simulink model "Target_Control_System"  (R2021b)
settings: Solver=FixedStepDiscrete  StartTime=0.0  StopTime=5  RelTol=1e-3
PreLoadFcn:
  | RTWConfigurationCB('preloadfcn', bdroot);
PostLoadFcn:
  | load('configuration/data_struct.mat');
  | load('configuration/fluxMaps_propMotor.mat');
  | load('configuration/parameterInit_PROP.mat');
  | load('configuration/parameterInit_PUMP.mat');
  | load('configuration/parameterInit_PITCH.mat');
  | load('configuration/parameterInit_TILT.mat');
  | %load('configuration/base_workspace_signal_definition.mat');
  | %load('resolvedatastores_to_baseworkspace_for_faster_simulation.mat');
model workspace (MAT data in the model file):
  SIMULATION_OPTIONS : Simulink.Parameter (value not decoded)
  TARGET_CODE_GEN : Simulink.Parameter (value not decoded)
  TCS_SAMPLE_FREQ_HZ : Simulink.Parameter (value not decoded)
symbols that are objects in the model workspace (value not decoded): TARGET_CODE_GEN, TCS_SAMPLE_FREQ_HZ
undefined symbols (not defined in the file): A_DQ_REF_LPF_INIT__PITCH, A_DQ_REF_LPF_INIT__PROP, A_DQ_REF_LPF_INIT__PUMP, A_DQ_REF_LPF_INIT__TILT, A_OBSERVER_CONFIDENCE_INIT__PITCH, A_OBSERVER_CONFIDENCE_INIT__PROP, A_OBSERVER_CONFIDENCE_INIT__PUMP, A_OBSERVER_CONFIDENCE_INIT__TILT, ACTUATOR_MAX_ANGLE_TRIP__PITCH, ACTUATOR_MIN_ANGLE_TRIP__PITCH, ACTUATOR_POS_SENSOR_INV_DIRECTION__PITCH, ACTUATOR_POS_SENSOR_INV_DIRECTION__TILT, ACTUATOR_POS_SENSOR_OFFSET__PITCH, ACTUATOR_POS_SENSOR_OFFSET__TILT, ADC_scaler1_baseaddr_TILT, ADC_SCALER_FLOAT_TO_FIXPOINT_EXPANSION, ANGLE_ELEC_FROM_SENSOR_OFFSET_INIT__PITCH, ANGLE_ELEC_FROM_SENSOR_OFFSET_INIT__PROP, ANGLE_ELEC_FROM_SENSOR_OFFSET_INIT__PUMP, ANGLE_ELEC_FROM_SENSOR_OFFSET_INIT__TILT, AUTO_CLEAR_FAULTS_ENABLED__PITCH, AUTO_CLEAR_FAULTS_ENABLED__PROP, AUTO_CLEAR_FAULTS_ENABLED__PUMP, AUTO_CLEAR_FAULTS_ENABLED__TILT, AUTO_CLEAR_FAULTS_WAIT_TICKS__PITCH, AUTO_CLEAR_FAULTS_WAIT_TICKS__PROP, AUTO_CLEAR_FAULTS_WAIT_TICKS__PUMP, AUTO_CLEAR_FAULTS_WAIT_TICKS__TILT, AUTO_I_ZERO_IDLE_TICKS__PITCH, AUTO_I_ZERO_IDLE_TICKS__PROP, AUTO_I_ZERO_IDLE_TICKS__PUMP, AUTO_I_ZERO_IDLE_TICKS__TILT, AUTO_I_ZERO_OFFSET_IDC_THRESHOLD__PITCH, AUTO_I_ZERO_OFFSET_IDC_THRESHOLD__PROP, AUTO_I_ZERO_OFFSET_IDC_THRESHOLD__PUMP, AUTO_I_ZERO_OFFSET_IDC_THRESHOLD__TILT, AUTO_I_ZERO_OFFSET_IPH_THRESHOLD__PITCH, AUTO_I_ZERO_OFFSET_IPH_THRESHOLD__PROP, AUTO_I_ZERO_OFFSET_IPH_THRESHOLD__PUMP, AUTO_I_ZERO_OFFSET_IPH_THRESHOLD__TILT, AUTO_SENSORLESS_SWITCHOVER_DISABLE_OMEGA, AUTO_SENSORLESS_SWITCHOVER_ENABLE_OMEGA, AUTO_SENSORLESS_SWITCHOVER_MIN_CONFIDENCE, AUXILIARY_PROTECTION_UNIT_BASEADDR__TILT, blanking_max_error_omega_INIT_PITCH, blanking_max_error_omega_INIT_TILT, blanking_max_error_position_INIT_PITCH, blanking_max_error_position_INIT_TILT, BRUTE_START_I_Q_REF_RAMP_SPEED__PITCH, BRUTE_START_I_Q_REF_RAMP_SPEED__PROP, BRUTE_START_I_Q_REF_RAMP_SPEED__PUMP, BRUTE_START_I_Q_REF_RAMP_SPEED__TILT, CONTROL_LOOP_DT_INIT__PITCH, CONTROL_LOOP_DT_INIT__PROP, CONTROL_LOOP_DT_INIT__PUMP, CONTROL_LOOP_DT_INIT__TILT, CORRECTION_FILTER_SCALE__PITCH, CORRECTION_FILTER_SCALE__PROP, CORRECTION_FILTER_SCALE__PUMP, CORRECTION_FILTER_SCALE__TILT ... (+458)
libraries: simulink x178, Reusables_Lib x24
(part 15 of 47)

== system Target_Control_System/Target_Control_System/MainLoop/pumpMotor_mainLoop/motorTaskMainFastStep(&oPump)/Lowpass Filtered Quantities for External World - Pump ==
  note: Low-pass filtered quantities for external world
  lpfQuantities : TriggerPort  TriggerType=function-call  VariantControl=Variant
  Constant1 : Constant  Value=0.00008  OutDataTypeStr=single  SampleTime=-1
  Data Store Read101 : DataStoreRead  DataStoreName=oPump  DataStoreElements=oPump.oMot_.oOut_.fIdLpf_  IndexOptions=Index vector (dialog)  Indices=1  OutputSizes=1
  Data Store Read102 : DataStoreRead  DataStoreName=oPump  DataStoreElements=oPump.oMot_.oOut_.fIqLpf_  IndexOptions=Index vector (dialog)  Indices=1  OutputSizes=1
  Data Store Read103 : DataStoreRead  DataStoreName=oPump  DataStoreElements=oPump.oMot_.oIn_.oAdcData_.fUdc_  IndexOptions=Index vector (dialog)  Indices=1  OutputSizes=1
  Data Store Read107 : DataStoreRead  DataStoreName=oPump  DataStoreElements=oPump.oMot_.oOut_.fUdcLpf_  IndexOptions=Index vector (dialog)  Indices=1  OutputSizes=1
  Data Store Read108 : DataStoreRead  DataStoreName=oPump  DataStoreElements=oPump.oMot_.oIn_.oAdcData_.fIdc_  IndexOptions=Index vector (dialog)  Indices=1  OutputSizes=1
  Data Store Read109 : DataStoreRead  DataStoreName=oPump  DataStoreElements=oPump.oMot_.oOut_.fIdcLpf_  IndexOptions=Index vector (dialog)  Indices=1  OutputSizes=1
  Data Store Read110 : DataStoreRead  DataStoreName=oPump  DataStoreElements=oPump.oMot_.oIn_.fPowerDc_  IndexOptions=Index vector (dialog)  Indices=1  OutputSizes=1
  Data Store Read111 : DataStoreRead  DataStoreName=oPump  DataStoreElements=oPump.oMot_.oOut_.fPowerDcLpf_  IndexOptions=Index vector (dialog)  Indices=1  OutputSizes=1
  Data Store Read112 : DataStoreRead  DataStoreName=oPump  DataStoreElements=oPump.oMot_.oOut_.fTEstimateLpf_  IndexOptions=Index vector (dialog)  Indices=1  OutputSizes=1
  Data Store Read113 : DataStoreRead  DataStoreName=oPump  DataStoreElements=oPump.oMot_.oState_.oRampDataIqRef_.fRampOut_  IndexOptions=Index vector (dialog)  Indices=1  OutputSizes=1
  Data Store Read114 : DataStoreRead  DataStoreName=oPump  DataStoreElements=oPump.oMot_.oOut_.fIqRefRampOutLpf_  IndexOptions=Index vector (dialog)  Indices=1  OutputSizes=1
  Data Store Read115 : DataStoreRead  DataStoreName=oPump  DataStoreElements=oPump.oMot_.oParam_.fADqRefLpf_  IndexOptions=Index vector (dialog)  Indices=1  OutputSizes=1
  Data Store Read116 : DataStoreRead  DataStoreName=oPump  DataStoreElements=oPump.oMot_.oIn_.fIdRefTotal_  IndexOptions=Index vector (dialog)  Indices=1  OutputSizes=1
  Data Store Read117 : DataStoreRead  DataStoreName=oPump  DataStoreElements=oPump.oMot_.oOut_.fIdRefLpf_  IndexOptions=Index vector (dialog)  Indices=1  OutputSizes=1
  Data Store Read118 : DataStoreRead  DataStoreName=oPump  DataStoreElements=oPump.oMot_.oIn_.fUqRef_  IndexOptions=Index vector (dialog)  Indices=1  OutputSizes=1
  Data Store Read119 : DataStoreRead  DataStoreName=oPump  DataStoreElements=oPump.oMot_.oOut_.fUqRefLpf_  IndexOptions=Index vector (dialog)  Indices=1  OutputSizes=1
  Data Store Read120 : DataStoreRead  DataStoreName=oPump  DataStoreElements=oPump.oMot_.oIn_.fUdRef_  IndexOptions=Index vector (dialog)  Indices=1  OutputSizes=1
  Data Store Read121 : DataStoreRead  DataStoreName=oPump  DataStoreElements=oPump.oMot_.oOut_.fUdRefLpf_  IndexOptions=Index vector (dialog)  Indices=1  OutputSizes=1
  Data Store Read17 : DataStoreRead  DataStoreName=oPump  DataStoreElements=oPump.oMot_.oIn_.fId_  IndexOptions=Index vector (dialog)  Indices=1  OutputSizes=1
  Data Store Read24 : DataStoreRead  DataStoreName=oPump  DataStoreElements=oPump.oMot_.oIn_.fIq_  IndexOptions=Index vector (dialog)  Indices=1  OutputSizes=1
  Data Store Read53 : DataStoreRead  DataStoreName=oPump  DataStoreElements=oPump.oMot_.oIn_.fTEstimate_  IndexOptions=Index vector (dialog)  Indices=1  OutputSizes=1
  Data Store Read88 : DataStoreRead  DataStoreName=oPump  DataStoreElements=oPump.oMot_.oOut_.fPowerDcLpf_  IndexOptions=Index vector (dialog)  Indices=1  OutputSizes=1
  Data Store Read89 : DataStoreRead  DataStoreName=oPump  DataStoreElements=oPump.oMot_.oOut_.fPowerDcXlpf_  IndexOptions=Index vector (dialog)  Indices=1  OutputSizes=1
  Data Store Read90 : DataStoreRead  DataStoreName=oPump  DataStoreElements=oPump.oMot_.oIn_.fOmegaEObserverLpf2_  IndexOptions=Index vector (dialog)  Indices=1  OutputSizes=1
  Data Store Read91 : DataStoreRead  DataStoreName=oPump  DataStoreElements=oPump.oMot_.oOut_.fOmegaEObserverXlpf2_  IndexOptions=Index vector (dialog)  Indices=1  OutputSizes=1
  Data Store Read96 : DataStoreRead  DataStoreName=oPump  DataStoreElements=oPump.oMot_.oParam_.fAOmegaXfilter2_  IndexOptions=Index vector (dialog)  Indices=1  OutputSizes=1
  Data Store Read97 : DataStoreRead  DataStoreName=oPump  DataStoreElements=oPump.oMot_.oParam_.fSlowPassFactor_  IndexOptions=Index vector (dialog)  Indices=1  OutputSizes=1
  Data Store Read98 : DataStoreRead  DataStoreName=oPump  DataStoreElements=oPump.oMot_.oIn_.fIPhaseMagnitude_  IndexOptions=Index vector (dialog)  Indices=1  OutputSizes=1
  Data Store Read99 : DataStoreRead  DataStoreName=oPump  DataStoreElements=oPump.oMot_.oState_.fIPhaseMagnitudeLpf_  IndexOptions=Index vector (dialog)  Indices=1  OutputSizes=1
  Data Store Write2 : DataStoreWrite  DataStoreName=oPump  DataStoreElements=oPump.oMot_.oOut_.fPowerDcXlpf_  IndexOptions=Index vector (dialog)  Indices=1  OutputSizes=1
  Data Store Write29 : DataStoreWrite  DataStoreName=oPump  DataStoreElements=oPump.oMot_.oOut_.fIdLpf_  IndexOptions=Index vector (dialog)  Indices=1  OutputSizes=1
  Data Store Write3 : DataStoreWrite  DataStoreName=oPump  DataStoreElements=oPump.oMot_.oState_.fIPhaseMagnitudeLpf_  IndexOptions=Index vector (dialog)  Indices=1  OutputSizes=1
  Data Store Write34 : DataStoreWrite  DataStoreName=oPump  DataStoreElements=oPump.oMot_.oOut_.fIqLpf_  IndexOptions=Index vector (dialog)  Indices=1  OutputSizes=1
  Data Store Write37 : DataStoreWrite  DataStoreName=oPump  DataStoreElements=oPump.oMot_.oOut_.fUdcLpf_  IndexOptions=Index vector (dialog)  Indices=1  OutputSizes=1
  Data Store Write38 : DataStoreWrite  DataStoreName=oPump  DataStoreElements=oPump.oMot_.oOut_.fIdcLpf_  IndexOptions=Index vector (dialog)  Indices=1  OutputSizes=1
  Data Store Write39 : DataStoreWrite  DataStoreName=oPump  DataStoreElements=oPump.oMot_.oOut_.fPowerDcLpf_  IndexOptions=Index vector (dialog)  Indices=1  OutputSizes=1
  Data Store Write40 : DataStoreWrite  DataStoreName=oPump  DataStoreElements=oPump.oMot_.oOut_.fTEstimateLpf_  IndexOptions=Index vector (dialog)  Indices=1  OutputSizes=1
  Data Store Write41 : DataStoreWrite  DataStoreName=oPump  DataStoreElements=oPump.oMot_.oOut_.fOmegaEObserverXlpf2_  IndexOptions=Index vector (dialog)  Indices=1  OutputSizes=1
  Data Store Write42 : DataStoreWrite  DataStoreName=oPump  DataStoreElements=oPump.oMot_.oOut_.fIqRefRampOutLpf_  IndexOptions=Index vector (dialog)  Indices=1  OutputSizes=1
  Data Store Write45 : DataStoreWrite  DataStoreName=oPump  DataStoreElements=oPump.oMot_.oOut_.fIdRefLpf_  IndexOptions=Index vector (dialog)  Indices=1  OutputSizes=1
  Data Store Write46 : DataStoreWrite  DataStoreName=oPump  DataStoreElements=oPump.oMot_.oOut_.fUqRefLpf_  IndexOptions=Index vector (dialog)  Indices=1  OutputSizes=1
  Data Store Write47 : DataStoreWrite  DataStoreName=oPump  DataStoreElements=oPump.oMot_.oOut_.fUdRefLpf_  IndexOptions=Index vector (dialog)  Indices=1  OutputSizes=1
  Divide{8..20} (13 alike) : Product  Inputs=**
  Sum{4..5,7,10..11,13,15,18,20..22,25,29} (13 alike) : Sum  Inputs=|+-
  Sum{3,6,8..9,12,14,16..17,19,24,26,30..31} (13 alike) : Sum  Inputs=|++
  wires:
  Data Store Read89/1 -> Sum24/2, Sum21/2
  Data Store Read117/1 -> Sum20/2, Sum19/2
  Sum10/1 -> Divide13/2
  Data Store Read98/1 -> Sum7/1
  Divide19/1 -> Sum31/1
  Data Store Read119/1 -> Sum29/2, Sum30/2
  Sum15/1 -> Divide14/2
  Sum30/1 -> Data Store Write46/1
  Data Store Read88/1 -> Sum21/1
  Data Store Read121/1 -> Sum25/2, Sum31/2
  Data Store Read116/1 -> Sum20/1
  Divide8/1 -> Sum3/1
  Sum7/1 -> Divide8/2
  Sum20/1 -> Divide16/2
  Data Store Read110/1 -> Sum11/1
  Divide9/1 -> Sum6/1
  Data Store Read111/1 -> Sum14/2, Sum11/2
  Sum21/1 -> Divide20/2
  Sum25/1 -> Divide19/2
  Sum29/1 -> Divide17/2
  Sum5/1 -> Divide10/2
  Data Store Read115/1 -> Divide15/1, Divide16/1, Divide19/1, Divide17/1
  Sum11/1 -> Divide11/2
  Data Store Read109/1 -> Sum12/2, Sum10/2
  Sum31/1 -> Data Store Write47/1
  Divide15/1 -> Sum17/1
  Data Store Read108/1 -> Sum10/1
  Divide18/1 -> Sum26/1
  Data Store Read99/1 -> Sum7/2, Sum3/2
  Sum8/1 -> Data Store Write34/1
  Sum13/1 -> Divide12/2
  Data Store Read97/1 -> Divide8/1, Divide9/1, Divide10/1, Divide12/1, Divide13/1, Divide14/1, Divide11/1
  Sum3/1 -> Data Store Write3/1
  Sum26/1 -> Data Store Write41/1
  Sum6/1 -> Data Store Write29/1
  Data Store Read112/1 -> Sum16/2, Sum15/2
  Divide17/1 -> Sum30/1
  Data Store Read90/1 -> Sum22/1
  Sum14/1 -> Data Store Write39/1
  Data Store Read102/1 -> Sum5/2, Sum8/2
  Data Store Read118/1 -> Sum29/1
  Sum9/1 -> Data Store Write37/1
  Sum18/1 -> Divide15/2
  Divide14/1 -> Sum16/1
  Sum22/1 -> Divide18/2
  Sum19/1 -> Data Store Write45/1
  Sum4/1 -> Divide9/2
  Sum12/1 -> Data Store Write38/1
  Data Store Read120/1 -> Sum25/1
  Sum17/1 -> Data Store Write42/1
  Divide12/1 -> Sum9/1
  Data Store Read91/1 -> Sum26/2, Sum22/2
  Divide10/1 -> Sum8/1
  Constant1/1 -> Divide20/1
  Data Store Read17/1 -> Sum4/1
  Data Store Read107/1 -> Sum9/2, Sum13/2
  Divide13/1 -> Sum12/1
  Data Store Read113/1 -> Sum18/1
  Data Store Read53/1 -> Sum15/1
  Data Store Read24/1 -> Sum5/1
  Divide20/1 -> Sum24/1
  Data Store Read103/1 -> Sum13/1
  Data Store Read101/1 -> Sum4/2, Sum6/2
  Data Store Read96/1 -> Divide18/1
  Divide16/1 -> Sum19/1
  Data Store Read114/1 -> Sum18/2, Sum17/2
  Sum24/1 -> Data Store Write2/1
  Sum16/1 -> Data Store Write40/1
  Divide11/1 -> Sum14/1

== system Target_Control_System/Target_Control_System/MainLoop/pumpMotor_mainLoop/motorTaskMainFastStep(&oPump)/Observer Confidence - Pump ==
  note: Observer confidence
      | // Two contributions, each adding 1/3 to give a value in range 0.0-1.0:
      | 	//  1. Magnitude of estimated flux relative to nominal flux (perhaps not for induction motors)
      | 	//  2. The relative noise on the estimated speed
  observerConfidence : TriggerPort  TriggerType=function-call  VariantControl=Variant
  Abs2 : Abs  OutDataTypeStr=single
  Abs3 : Abs  OutDataTypeStr=single
  Abs5 : Abs  OutDataTypeStr=single
  Add10 : Sum  Inputs=|-+
  Add11 : Sum
  Add2 : Sum  Inputs=+-
  Add7 : Sum  Inputs=|+-
  Add8 : Sum  Inputs=|-+
  Add9 : Sum  Inputs=|-+
  Constant14 : Constant  OutDataTypeStr=single  SampleTime=-1
  Data Store Read1 : DataStoreRead  DataStoreName=oPump  DataStoreElements=oPump.oMot_.oParam_.fAObserverConfidence_  IndexOptions=Index vector (dialog)  Indices=1  OutputSizes=1
  Data Store Read37 : DataStoreRead  DataStoreName=oPump  DataStoreElements=oPump.oMot_.oIn_.fOmegaEObserverLpf2_  IndexOptions=Index vector (dialog)  Indices=1  OutputSizes=1
  Data Store Read4 : DataStoreRead  DataStoreName=oPump  DataStoreElements=oPump.oMot_.oIn_.fFluxMainMagnitudeLpf_  IndexOptions=Index vector (dialog)  Indices=1  OutputSizes=1
  Data Store Read61 : DataStoreRead  DataStoreName=oPump  DataStoreElements=oPump.oMot_.oIn_.fOmegaEObserverRaw2_  IndexOptions=Index vector (dialog)  Indices=1  OutputSizes=1
  Data Store Read83 : DataStoreRead  DataStoreName=oPump  DataStoreElements=oPump.oMot_.oParam_.fMainFluxNominal_  IndexOptions=Index vector (dialog)  Indices=1  OutputSizes=1
  Data Store Write33 : DataStoreWrite  DataStoreName=oPump  DataStoreElements=oPump.oMot_.oState_.fObserverConfidence_  IndexOptions=Index vector (dialog)  Indices=1  OutputSizes=1
  Divide1 : Product  Inputs=*/
  Divide2 : Product  Inputs=*/
  Gain11 : Gain  Gain=0.83
  Gain5 : Gain  Gain=0.4
  Half : Constant  Value=0.5  OutDataTypeStr=single  SampleTime=-1
  Half1 : Constant  Value=0.5  OutDataTypeStr=single  SampleTime=-1
  IIR : Subsystem
  Saturation2 : Saturate  UpperLimit=1.25  LowerLimit=-inf
  Saturation3 : Saturate  UpperLimit=0.6  LowerLimit=-inf
  Switch3 : Switch  Criteria=u2 > Threshold  Threshold=0.5
  Zero0 : Constant  Value=0  OutDataTypeStr=single  SampleTime=-1
  isNaN : RelationalOperator  Operator=isNaN  OutDataTypeStr=boolean  RndMeth=Simplest
  wires:
  Saturation2/1 -> Gain5/1
  Switch3/1 -> IIR/1(In)
  Data Store Read4/1 -> Add7/1
  Half1/1 -> Add10/2
  Saturation3/1 -> Gain11/1
  Constant14/1 -> Add2/1
  IIR/1(Out) -> Data Store Write33/1
  Add9/1 -> Abs3/1
  Data Store Read61/1 -> Add9/1
  Data Store Read83/1 -> Divide1/2, Add7/2
  Add11/1 -> isNaN/1, Switch3/3  "fObserverConfidence_"
  Abs2/1 -> Divide1/1
  isNaN/1 -> Switch3/2
  Half/1 -> Add8/2
  Zero0/1 -> Switch3/1
  Data Store Read37/1 -> Add9/2, Abs5/1
  Add10/1 -> Add11/2
  Add8/1 -> Add11/1
  Data Store Read1/1 -> IIR/3(K), Add2/2
  Divide2/1 -> Saturation3/1
  Abs5/1 -> Divide2/2
  Gain11/1 -> Add10/1
  Add7/1 -> Abs2/1
  Gain5/1 -> Add8/1
  Divide1/1 -> Saturation2/1
  Add2/1 -> IIR/2(1-K)
  Abs3/1 -> Divide2/1

== system Target_Control_System/Target_Control_System/MainLoop/pumpMotor_mainLoop/motorTaskMainFastStep(&oPump)/PWM for Simulation ==
  Enable : EnablePort
  Constant : Constant  OutDataTypeStr=uint32  SampleTime=-1
  Constant1 : Constant  Value=0  OutDataTypeStr=uint32  SampleTime=-1
  Data Store Read1 : DataStoreRead  DataStoreName=oPump  DataStoreElements=oPump.oIsr_.oState_.iPwmUpdated_  IndexOptions=Index vector (dialog)  Indices=1  OutputSizes=1
  Data Store Write18 : DataStoreWrite  DataStoreName=oPump  DataStoreElements=oPump.oIsr_.oOut_.uiPwmSetByIsr_  IndexOptions=Index vector (dialog)  Indices=1  OutputSizes=1
  NOT : Logic  Operator=NOT  AllPortsSameDT=off  OutDataTypeStr=boolean
  Scope : Scope
  Subsystem : Subsystem
  Subsystem1 : Subsystem
  Switch1 : Switch  Criteria=u2 > Threshold
  Switch2 : Switch  Criteria=u2 > Threshold
  Motor : Outport
  wires:
  NOT/1 -> Subsystem1/Enable
  Subsystem1/1(pumpMotor_PWMticks) -> Switch1/3
  Subsystem/1(pumpMotor_PWMticks) -> Switch1/1
  Constant1/1 -> Switch2/3
  Constant/1 -> Switch2/1
  Switch2/1 -> Data Store Write18/1
  Switch1/1 -> Motor/1  "pumpMotor_PWMticks"
  Data Store Read1/1 -> Subsystem/Enable, Switch1/2, NOT/1, Scope/1, Switch2/2

== system Target_Control_System/Target_Control_System/MainLoop/pumpMotor_mainLoop/motorTaskMainFastStep(&oPump)/Variant Subsystem ==
  note: 1) Add Subsystem or Model blocks as valid variant choices.
      | 2) You cannot connect blocks at this level. At simulation, connectivity is automatically
      | determined, based on the active variant and port name matching.
  Target_Code_Gen_0 : Subsystem  VariantControl=(default)
  Target_Code_Gen_1 : Subsystem  VariantControl=TARGET_CODE_GEN==1
  Output : Outport

== system Target_Control_System/Target_Control_System/MainLoop/pumpMotor_mainLoop/motorTaskMainFastStep(&oPump)/motorTaskManagePwmRequestFlags() ==
  motorTaskManagePwmRequestFlags : TriggerPort  TriggerType=function-call  VariantControl=Variant
  Constant : Constant  Value=0  OutDataTypeStr=uint32  SampleTime=-1
  Data Store Read : DataStoreRead  DataStoreName=oPump  DataStoreElements=oPump.oMot_.oIn_.uiPwmSetByIsr_  IndexOptions=Index vector (dialog)  Indices=1  OutputSizes=1
  Data Store Read1 : DataStoreRead  DataStoreName=oPump  DataStoreElements=oPump.oMot_.oOut_.uiPwmRequestFromMain_  IndexOptions=Index vector (dialog)  Indices=1  OutputSizes=1
  Data Store Write : DataStoreWrite  DataStoreName=oPump  DataStoreElements=oPump.oMot_.oOut_.uiPwmRequestFromMain_  IndexOptions=Index vector (dialog)  Indices=1  OutputSizes=1
  Switch : Switch  Criteria=u2 > Threshold  OutDataTypeStr=uint32
  wires:
  Data Store Read1/1 -> Switch/3
  Constant/1 -> Switch/1
  Switch/1 -> Data Store Write/1
  Data Store Read/1 -> Switch/2

== system Target_Control_System/Target_Control_System/MainLoop/pumpMotor_mainLoop/motorTaskMainFastStep(&oPump)/resetFlag_uiDataFromIsrToMainUpdated ==
  resetFlag_uiDataFromIsrToMainUpdated : TriggerPort  TriggerType=function-call  VariantControl=Variant
  Constant : Constant  Value=0  OutDataTypeStr=uint32  SampleTime=-1
  Data Store Write9 : DataStoreWrite  DataStoreName=oPump  DataStoreElements=oPump.oMot_.oIn_.uiDataFromIsrToMainUpdated_  IndexOptions=Index vector (dialog)  Indices=1  OutputSizes=1
  wires:
  Constant/1 -> Data Store Write9/1

== system Target_Control_System/Target_Control_System/MainLoop/tiltMotor_mainLoop/Decimation gate for 10 Hz Tilt/Function-Call Subsystem ==
  motorTaskMainDecimationBStep : TriggerPort  TriggerType=function-call  VariantControl=Variant
  DC_overvoltage : Stateflow chart  TreatAsAtomicUnit=on
  Dynamic_current_limiting : Subsystem

== system Target_Control_System/Target_Control_System/MainLoop/tiltMotor_mainLoop/Decimation gate for 200 Hz Tilt/motorTaskMainDecimationAStep(&oTilt) ==
  motorTaskMainDecimationAStep : TriggerPort  TriggerType=function-call  VariantControl=Variant
  Check zero current if inverter off : Subsystem  TreatAsAtomicUnit=on
  Current control inactive : Subsystem  TreatAsAtomicUnit=on
  Current offset nulling : Subsystem  TreatAsAtomicUnit=on
  DClink_overCurrentProtection : Subsystem  TreatAsAtomicUnit=on
  Forced current injection for broken input sensors : Subsystem  Commented=on  TreatAsAtomicUnit=on
  Function-Call Generator : simulink/Ports & Subsystems/Function-Call Generator  sample_time=-1  numberOfIterations=1  DisallowWideOutput=off
  Function-Call Split{1..5,10} (6 alike) : FunctionCallSplit  NumOutputPorts=2
  Idle controller : Subsystem  TreatAsAtomicUnit=on
  Position control checks : Subsystem  TreatAsAtomicUnit=on
  wires:
  Function-Call Split1/2 -> Function-Call Split2/1
  Function-Call Split3/2 -> Function-Call Split4/1
  Function-Call Split4/2 -> Function-Call Split5/1
  Function-Call Split2/2 -> Function-Call Split3/1
  Function-Call Generator/1 -> Function-Call Split10/1
  Function-Call Split4/1 -> Forced current injection for broken input sensors/Trigger
  Function-Call Split3/1 -> Current control inactive/Trigger
  Function-Call Split1/1 -> Check zero current if inverter off/Trigger
  Function-Call Split10/2 -> Function-Call Split1/1
  Function-Call Split5/1 -> Idle controller/Trigger
  Function-Call Split2/1 -> Current offset nulling/Trigger
  Function-Call Split5/2 -> Position control checks/Trigger
  Function-Call Split10/1 -> DClink_overCurrentProtection/Trigger

== system Target_Control_System/Target_Control_System/MainLoop/tiltMotor_mainLoop/Decimation gate for 5000 Hz Tilt/motorTaskProcessExternalSetpoints(&oTilt) ==
  note: // Do not set certain variables during auto forced angle start or resistance measurement // This whole code below should be cleaned up, probably a switch case tied to the state machine.
      | // The different modes, (position control, speed control, current control) should get different state numbers to facilitate this.
  note: // Take externally requested setpoints (already set in the 'in' struct) and apply them (after sanitizing) to the right place in the control loop, also depending on the state that the drive is in.
  motorTaskProcessExternalSetpoints : TriggerPort  TriggerType=function-call  VariantControl=Variant
  Function-Call Generator : simulink/Ports & Subsystems/Function-Call Generator  sample_time=-1  numberOfIterations=1  DisallowWideOutput=off
  Function-Call Split1 : FunctionCallSplit  NumOutputPorts=2
  Function-Call Split10 : FunctionCallSplit  NumOutputPorts=2
  hot_standby : Subsystem
  passive_holding_mode : Subsystem
  set_target : Subsystem
  wires:
  Function-Call Split1/2 -> set_target/Trigger
  Function-Call Split10/2 -> Function-Call Split1/1
  Function-Call Split1/1 -> hot_standby/Trigger
  Function-Call Split10/1 -> passive_holding_mode/Trigger
  Function-Call Generator/1 -> Function-Call Split10/1

== system Target_Control_System/Target_Control_System/MainLoop/tiltMotor_mainLoop/mainTask_tilt/PWM for Simulation ==
  Enable : EnablePort
  Bus Creator3 : BusCreator  Inputs=3
  Constant : Constant  OutDataTypeStr=uint32  SampleTime=-1
  Constant{1..4} (4 alike) : Constant  Value=0  OutDataTypeStr=uint32  SampleTime=-1
  Data Store Read1 : DataStoreRead  DataStoreName=oTilt  DataStoreElements=oTilt.oIsr_.oState_.iPwmUpdated_  IndexOptions=Index vector (dialog)  Indices=1  OutputSizes=1
  Data Store Read9 : DataStoreRead  DataStoreName=oTilt  DataStoreElements=oTilt.oMot_.oOut_.uiEnableGateDrive_  IndexOptions=Index vector (dialog)  Indices=1  OutputSizes=1
  Data Store Write18 : DataStoreWrite  DataStoreName=oTilt  DataStoreElements=oTilt.oIsr_.oOut_.uiPwmSetByIsr_  IndexOptions=Index vector (dialog)  Indices=1  OutputSizes=1
  NOT : Logic  Operator=NOT  AllPortsSameDT=off  OutDataTypeStr=boolean
  Scope : Scope
  Subsystem : Subsystem
  Subsystem1 : Subsystem
  Switch1 : Switch  Criteria=u2 > Threshold
  Switch2 : Switch  Criteria=u2 > Threshold
  Switch3 : Switch  Criteria=u2 > Threshold
  Out1 : Outport
  wires:
  Subsystem/1(tiltMotor_PWMticks) -> Switch2/1
  Switch2/1 -> Switch1/1
  Switch3/1 -> Data Store Write18/1
  Constant4/1 -> Switch3/3
  Data Store Read1/1 -> Subsystem/Enable, Switch2/2, NOT/1, Scope/1, Switch3/2
  NOT/1 -> Subsystem1/Enable
  Subsystem1/1(tiltMotor_PWMticks) -> Switch2/3
  Constant/1 -> Switch3/1
  Constant1/1 -> Bus Creator3/1  "Aticks"
  Bus Creator3/1 -> Switch1/3
  Switch1/1 -> Out1/1  "tiltMotor_PWMticks"
  Constant3/1 -> Bus Creator3/3  "Cticks"
  Data Store Read9/1 -> Switch1/2
  Constant2/1 -> Bus Creator3/2  "Bticks"

== system Target_Control_System/Target_Control_System/MainLoop/tiltMotor_mainLoop/mainTask_tilt/Variant Subsystem ==
  note: 1) Add Subsystem or Model blocks as valid variant choices.
      | 2) You cannot connect blocks at this level. At simulation, connectivity is automatically
      | determined, based on the active variant and port name matching.
  Target_Code_Gen_0 : Subsystem  VariantControl=(default)
  Target_Code_Gen_1 : Subsystem  VariantControl=TARGET_CODE_GEN==1
  Out1 : Outport

== system Target_Control_System/Target_Control_System/MainLoop/tiltMotor_mainLoop/mainTask_tilt/motorTaskMainFastStep(&oTilt) ==
  function : TriggerPort  TriggerType=function-call  VariantControl=Variant
  Automatic switching to sensorless - Tilt : Subsystem  Commented=on
  Control Loops - Tilt : Subsystem
  Correction Constants for Observer and Control - Tilt : Subsystem  Commented=on
  Function-Call Generator : simulink/Ports & Subsystems/Function-Call Generator  sample_time=-1  numberOfIterations=1  DisallowWideOutput=off
  Function-Call Split{1..6,10} (7 alike) : FunctionCallSplit  NumOutputPorts=2
  Lowpass Filtered Quantities for External World - Tilt : Subsystem
  Mechanical System - Tilt : Subsystem
  Motor Acceleration - Tilt : Subsystem
  Observer Confidence - Tilt : Subsystem  Commented=on
  Software Overcurrent Protection - Tilt : Subsystem
  enableDrive(&oTilt) : Stateflow chart  TreatAsAtomicUnit=on
  initiateOffsetNulling(&oTilt) : Stateflow chart  TreatAsAtomicUnit=on
  wires:
  Function-Call Split6/1 -> Correction Constants for Observer and Control - Tilt/Trigger
  Function-Call Split4/1 -> Lowpass Filtered Quantities for External World - Tilt/Trigger
  Function-Call Split4/2 -> Function-Call Split5/1
  Function-Call Split1/1 -> Mechanical System - Tilt/Trigger
  Function-Call Split3/2 -> Function-Call Split4/1
  Function-Call Split6/2 -> Motor Acceleration - Tilt/Trigger
  Function-Call Split5/2 -> Function-Call Split6/1
  Function-Call Split1/2 -> Function-Call Split2/1
  Function-Call Split3/1 -> Automatic switching to sensorless - Tilt/Trigger
  Function-Call Split2/2 -> Function-Call Split3/1
  Function-Call Split5/1 -> Control Loops - Tilt/Trigger
  Function-Call Split10/2 -> Function-Call Split1/1
  Function-Call Split10/1 -> Software Overcurrent Protection - Tilt/Trigger
  Function-Call Split2/1 -> Observer Confidence - Tilt/Trigger
  Function-Call Generator/1 -> Function-Call Split10/1

== system Target_Control_System/Target_Control_System/MainLoop/tiltMotor_mainLoop/mainTask_tilt/motorTaskManagePwmRequestFlags(&oTilt) ==
  motorTaskManagePwmRequestFlags : TriggerPort  TriggerType=function-call  VariantControl=Variant
  Constant : Constant  Value=0  OutDataTypeStr=uint32  SampleTime=-1
  Data Store Read : DataStoreRead  DataStoreName=oTilt  DataStoreElements=oTilt.oMot_.oIn_.uiPwmSetByIsr_  IndexOptions=Index vector (dialog)  Indices=1  OutputSizes=1
  Data Store Read1 : DataStoreRead  DataStoreName=oTilt  DataStoreElements=oTilt.oMot_.oOut_.uiPwmRequestFromMain_  IndexOptions=Index vector (dialog)  Indices=1  OutputSizes=1
  Data Store Write : DataStoreWrite  DataStoreName=oTilt  DataStoreElements=oTilt.oMot_.oOut_.uiPwmRequestFromMain_  IndexOptions=Index vector (dialog)  Indices=1  OutputSizes=1
  Switch : Switch  Criteria=u2 > Threshold  OutDataTypeStr=uint32
  wires:
  Data Store Read1/1 -> Switch/3
  Constant/1 -> Switch/1
  Switch/1 -> Data Store Write/1
  Data Store Read/1 -> Switch/2

== system Target_Control_System/Target_Control_System/MainLoop/tiltMotor_mainLoop/mainTask_tilt/resetFlag_uiDataFromIsrToMainUpdated ==
  resetFlag_uiDataFromIsrToMainUpdated : TriggerPort  TriggerType=function-call  VariantControl=Variant
  Constant : Constant  Value=0  OutDataTypeStr=uint32  SampleTime=-1
  Data Store Write : DataStoreWrite  DataStoreName=oTilt  DataStoreElements=oTilt.oMot_.oIn_.uiDataFromIsrToMainUpdated_  IndexOptions=Index vector (dialog)  Indices=1  OutputSizes=1
  wires:
  Constant/1 -> Data Store Write/1

== system Target_Control_System/Target_Control_System/Simulation Controls/Simulation Data Store Initialization/initializeDataForPitch()/initializeHardwareInvPitch() ==
  note: ***Not sure if these should be "...July2019..." for current boards or not.
  Constant : Constant  Value=I_TRIP_HW_INIT__PITCH  OutDataTypeStr=single  SampleTime=-1
  Constant1 : Constant  Value=DEADTIME_NS__PITCH  OutDataTypeStr=single  SampleTime=-1
  Constant10 : Constant  Value=VOLTAGE_OFFSET_DC_V_JULY2019__PITCH  OutDataTypeStr=single  SampleTime=-1
  Constant11 : Constant  Value=FULL_SCALE_VALUE_DC_VOLTAGE_V_JULY2019__PITCH  OutDataTypeStr=single  SampleTime=-1
  Constant12 : Constant  Value=ADC_SCALER_FLOAT_TO_FIXPOINT_EXPANSION  OutDataTypeStr=single  SampleTime=-1
  Constant13 : Constant  Value=PHASE_CURRENT_SUM_MAX_IMBALANCE__PITCH  OutDataTypeStr=single  SampleTime=-1
  Constant14 : Constant  Value=MAX_IDENTICAL_SAMPLES_PHASE_CURRENT__PITCH  OutDataTypeStr=int32  SampleTime=-1
  Constant2 : Constant  Value=IIR_DC_F_INIT__PITCH  OutDataTypeStr=single  SampleTime=-1
  Constant3 : Constant  Value=IIR_UPHASE_F_INIT__PITCH  OutDataTypeStr=single  SampleTime=-1
  Constant4 : Constant  Value=IIR_IPHASE_F_INIT__PITCH  OutDataTypeStr=single  SampleTime=-1
  Constant5 : Constant  Value=IIR_F_SAMPLE__PITCH  OutDataTypeStr=single  SampleTime=-1
  Constant6 : Constant  Value=FULL_SCALE_VALUE_PHASE_VOLTAGE_V__PITCH  OutDataTypeStr=single  SampleTime=-1
  Constant7 : Constant  Value=FULL_SCALE_VALUE_PHASE_CURRENT_A__PITCH  OutDataTypeStr=single  SampleTime=-1
  Constant8 : Constant  Value=FULL_SCALE_VALUE_DC_CURRENT_A__PITCH  OutDataTypeStr=single  SampleTime=-1
  Constant9 : Constant  Value=VOLTAGE_OFFSET_V__PITCH  OutDataTypeStr=single  SampleTime=-1
  Data Store Read : DataStoreRead  DataStoreName=oPitch  DataStoreElements=oPitch.oHw_.fFullScaleValuePhaseCurrent_  IndexOptions=Index vector (dialog)  Indices=1  OutputSizes=1
  Data Store Read1 : DataStoreRead  DataStoreName=oPitch  DataStoreElements=oPitch.oHw_.fFullScaleValueDcCurrent_  IndexOptions=Index vector (dialog)  Indices=1  OutputSizes=1
  Data Store Read2 : DataStoreRead  DataStoreName=oPitch  DataStoreElements=oPitch.oHw_.fFullScaleValuePhaseVoltage_  IndexOptions=Index vector (dialog)  Indices=1  OutputSizes=1
  Data Store Read3 : DataStoreRead  DataStoreName=oPitch  DataStoreElements=oPitch.oHw_.fFullScaleValueDcVoltage_  IndexOptions=Index vector (dialog)  Indices=1  OutputSizes=1
  Data Store Write : DataStoreWrite  DataStoreName=oPitch  DataStoreElements=oPitch.oHw_.fTripLimitHardware_  IndexOptions=Index vector (dialog)  Indices=1  OutputSizes=1
  Data Store Write1 : DataStoreWrite  DataStoreName=oPitch  DataStoreElements=oPitch.oHw_.fDeadtimeNs_  IndexOptions=Index vector (dialog)  Indices=1  OutputSizes=1
  Data Store Write10 : DataStoreWrite  DataStoreName=oPitch  DataStoreElements=oPitch.oHw_.fFullScaleValueDcVoltage_  IndexOptions=Index vector (dialog)  Indices=1  OutputSizes=1
  Data Store Write11 : DataStoreWrite  DataStoreName=oPitch  DataStoreElements=oPitch.oHw_.fVoltageOffsetDcInVolts_  IndexOptions=Index vector (dialog)  Indices=1  OutputSizes=1
  Data Store Write12 : DataStoreWrite  DataStoreName=oPitch  DataStoreElements=oPitch.oHw_.iScalePhaseCurrentLong_  IndexOptions=Index vector (dialog)  Indices=1  OutputSizes=1
  Data Store Write13 : DataStoreWrite  DataStoreName=oPitch  DataStoreElements=oPitch.oHw_.iScaleDcCurrentLong_  IndexOptions=Index vector (dialog)  Indices=1  OutputSizes=1
  Data Store Write14 : DataStoreWrite  DataStoreName=oPitch  DataStoreElements=oPitch.oHw_.iScalePhaseVoltageLong_  IndexOptions=Index vector (dialog)  Indices=1  OutputSizes=1
  Data Store Write15 : DataStoreWrite  DataStoreName=oPitch  DataStoreElements=oPitch.oHw_.iScaleDcVoltageLong_  IndexOptions=Index vector (dialog)  Indices=1  OutputSizes=1
  Data Store Write16 : DataStoreWrite  DataStoreName=oPitch  DataStoreElements=oPitch.oHw_.fPhaseCurrentSumMaxImbalance_  IndexOptions=Index vector (dialog)  Indices=1  OutputSizes=1
  Data Store Write17 : DataStoreWrite  DataStoreName=oPitch  DataStoreElements=oPitch.oHw_.iMaxIdenticalSamplesPhaseCurrent_  IndexOptions=Index vector (dialog)  Indices=1  OutputSizes=1
  Data Store Write2 : DataStoreWrite  DataStoreName=oPitch  DataStoreElements=oPitch.oHw_.fIirDcFInit_  IndexOptions=Index vector (dialog)  Indices=1  OutputSizes=1
  Data Store Write3 : DataStoreWrite  DataStoreName=oPitch  DataStoreElements=oPitch.oHw_.fIirUphaseFInit_  IndexOptions=Index vector (dialog)  Indices=1  OutputSizes=1
  Data Store Write4 : DataStoreWrite  DataStoreName=oPitch  DataStoreElements=oPitch.oHw_.fIirIphaseFInit_  IndexOptions=Index vector (dialog)  Indices=1  OutputSizes=1
  Data Store Write5 : DataStoreWrite  DataStoreName=oPitch  DataStoreElements=oPitch.oHw_.fIirFSample_  IndexOptions=Index vector (dialog)  Indices=1  OutputSizes=1
  Data Store Write6 : DataStoreWrite  DataStoreName=oPitch  DataStoreElements=oPitch.oHw_.fFullScaleValuePhaseCurrent_  IndexOptions=Index vector (dialog)  Indices=1  OutputSizes=1
  Data Store Write7 : DataStoreWrite  DataStoreName=oPitch  DataStoreElements=oPitch.oHw_.fFullScaleValueDcCurrent_  IndexOptions=Index vector (dialog)  Indices=1  OutputSizes=1
  Data Store Write8 : DataStoreWrite  DataStoreName=oPitch  DataStoreElements=oPitch.oHw_.fFullScaleValuePhaseVoltage_  IndexOptions=Index vector (dialog)  Indices=1  OutputSizes=1
  Data Store Write9 : DataStoreWrite  DataStoreName=oPitch  DataStoreElements=oPitch.oHw_.fVoltageOffsetInVolts_  IndexOptions=Index vector (dialog)  Indices=1  OutputSizes=1
  Divide{,1..3} (4 alike) : Product  Inputs=**  OutDataTypeStr=int32
  wires:
  Constant14/1 -> Data Store Write17/1
  Constant13/1 -> Data Store Write16/1
  Divide2/1 -> Data Store Write14/1
  Divide3/1 -> Data Store Write15/1
  Divide1/1 -> Data Store Write13/1
  Divide/1 -> Data Store Write12/1
  Constant12/1 -> Divide1/2, Divide/2, Divide2/2, Divide3/2
  Data Store Read3/1 -> Divide3/1
  Data Store Read2/1 -> Divide2/1
  Data Store Read1/1 -> Divide1/1
  Data Store Read/1 -> Divide/1
  Constant11/1 -> Data Store Write10/1
  Constant10/1 -> Data Store Write11/1
  Constant9/1 -> Data Store Write9/1
  Constant6/1 -> Data Store Write8/1
  Constant8/1 -> Data Store Write7/1
  Constant7/1 -> Data Store Write6/1
  Constant5/1 -> Data Store Write5/1
  Constant4/1 -> Data Store Write4/1
  Constant3/1 -> Data Store Write3/1
  Constant2/1 -> Data Store Write2/1
  Constant1/1 -> Data Store Write1/1
  Constant/1 -> Data Store Write/1
